simulink library "csu_cmt_convert_measured_temps_collection_lib"  (R2014b)
settings: Solver=ode45  StartTime=0.0  StopTime=10.0  RelTol=1e-3
libraries: util_info_lib x1
settings Model: Creator=escrane  LastModifiedBy=mstewart

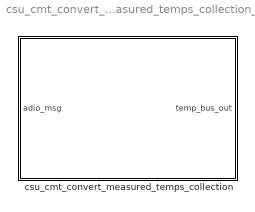
== system csu_cmt_convert_measured_temps_collection_lib ==
  csu_cmt_convert_measured_temps_collection : Subsystem

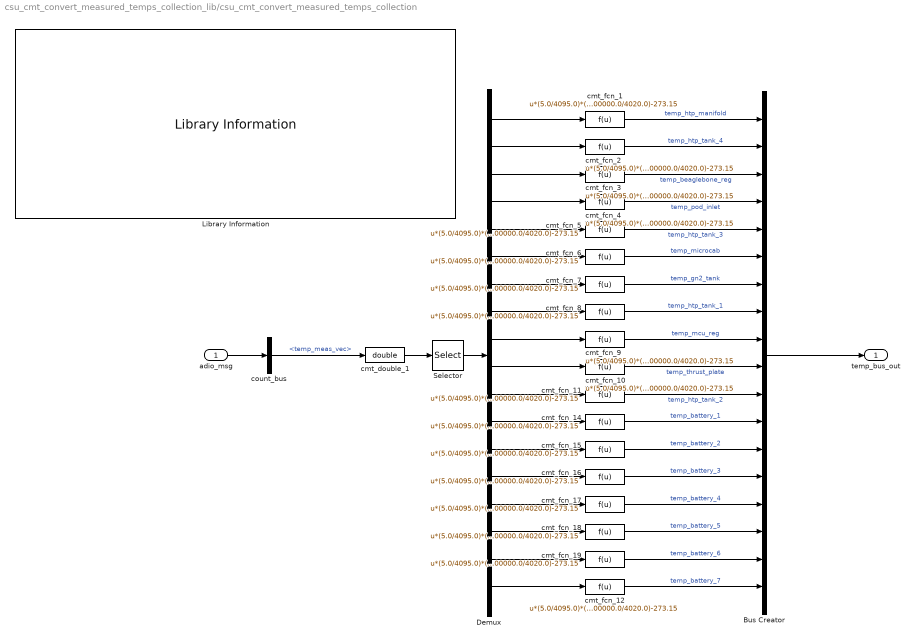
== system csu_cmt_convert_measured_temps_collection_lib/csu_cmt_convert_measured_temps_collection ==
  adio_msg : Inport
  Bus Creator : BusCreator  Inputs=18
  Demux : Demux  Outputs=18
  Library Information : util_info_lib/Library Information  owner='escrane'
  Selector : Selector  InputPortWidth=tcs_n_temps  Indices=tcs_temp_special_index_vector
  cmt_double_1 : DataTypeConversion  OutDataTypeStr=double
  cmt_fcn_{1..12,14..19} (18 alike) : Fcn  Expr=u*(5.0/4095.0)*(1000000.0/4020.0)-273.15
  count_bus : BusSelector  OutputSignals=temp_meas_vec
  temp_bus_out : Outport
  wires:
  cmt_fcn_19/1 -> Bus Creator/17  "temp_battery_6"
  cmt_fcn_18/1 -> Bus Creator/16  "temp_battery_5"
  cmt_fcn_17/1 -> Bus Creator/15  "temp_battery_4"
  cmt_fcn_14/1 -> Bus Creator/12  "temp_battery_1"
  cmt_fcn_15/1 -> Bus Creator/13  "temp_battery_2"
  cmt_fcn_12/1 -> Bus Creator/18  "temp_battery_7"
  cmt_fcn_16/1 -> Bus Creator/14  "temp_battery_3"
  Demux/12 -> cmt_fcn_14/1
  Demux/13 -> cmt_fcn_15/1
  Demux/17 -> cmt_fcn_19/1
  Demux/16 -> cmt_fcn_18/1
  Demux/14 -> cmt_fcn_16/1
  Demux/15 -> cmt_fcn_17/1
  Demux/18 -> cmt_fcn_12/1
  adio_msg/1 -> count_bus/1
  count_bus/1 -> cmt_double_1/1  "<temp_meas_vec>"
  cmt_double_1/1 -> Selector/1
  Selector/1 -> Demux/1
  Demux/1 -> cmt_fcn_1/1
  Demux/2 -> cmt_fcn_2/1
  Demux/3 -> cmt_fcn_3/1
  Demux/4 -> cmt_fcn_4/1
  Demux/6 -> cmt_fcn_6/1
  Demux/8 -> cmt_fcn_8/1
  Demux/5 -> cmt_fcn_5/1
  Demux/7 -> cmt_fcn_7/1
  Demux/10 -> cmt_fcn_10/1
  Demux/11 -> cmt_fcn_11/1
  Demux/9 -> cmt_fcn_9/1
  cmt_fcn_7/1 -> Bus Creator/7  "temp_gn2_tank"
  cmt_fcn_8/1 -> Bus Creator/8  "temp_htp_tank_1"
  cmt_fcn_6/1 -> Bus Creator/6  "temp_microcab"
  cmt_fcn_4/1 -> Bus Creator/4  "temp_pod_inlet"
  cmt_fcn_5/1 -> Bus Creator/5  "temp_htp_tank_3"
  cmt_fcn_3/1 -> Bus Creator/3  "temp_beaglebone_reg"
  cmt_fcn_10/1 -> Bus Creator/10  "temp_thrust_plate"
  cmt_fcn_11/1 -> Bus Creator/11  "temp_htp_tank_2"
  cmt_fcn_2/1 -> Bus Creator/2  "temp_htp_tank_4"
  Bus Creator/1 -> temp_bus_out/1
  cmt_fcn_1/1 -> Bus Creator/1  "temp_htp_manifold"
  cmt_fcn_9/1 -> Bus Creator/9  "temp_mcu_reg"
